simulink model "Simulation_Uncontrolled"  (R2020b)
settings: Solver=FixedStepAuto  StartTime=0.0  StopTime=8  FixedStep=0.01  RelTol=1e-3
undefined symbols (not defined in the file): sigbuilder_block
libraries: simulink x1
settings Model: Creator=Kacper  LastModifiedBy=Kacper

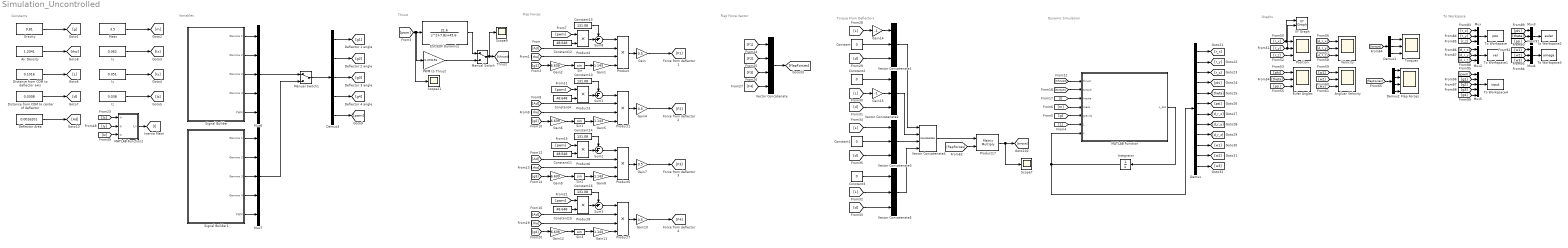
== system Simulation_Uncontrolled ==
  note: Graphs
  note: To Workspace
  note: Flap Force Vector
  note: Dynamic Simulation
  note: Torque From Deflectors
  note: Flap Forces
  note: Thrust
  note: Constants
  note: Variables
  Air Density : Constant  Value=1.2041
  Angluar Velocity : Scope  NumInputPorts=3
  Constant{,1..3} (4 alike) : Constant  Value=0
  Constant{10,13..14,16} (4 alike) : Constant  Value=131.08
  Constant{4,11..12,15} (4 alike) : Constant  Value=48.648
  Deflector Area : Constant  Value=0.0016201
  Demux : Demux  Outputs=12
  Demux1 : Demux  Outputs=3
  Demux2 : Demux
  Demux3 : Demux  Outputs=5
  Distance from COM to center of deflector : Constant  Value=0.0308
  Distance from COM to deflector axis : Constant  Value=0.1016
  ESC/EDF Dynamics : TransferFcn  Numerator=[21.6]  Denominator=[1 7.8 45.6]
  Euler Angles : Scope  NumInputPorts=3
  Flap Forces : Scope  NumInputPorts=4
  Gain{,4,7,10} (4 alike) : Gain  Gain=0.5
  Gain{1,5,8,11} (4 alike) : Gain  Gain=1.143
  Gain{2,6,9,12} (4 alike) : Gain  Gain=6.639
  Gain14 : Gain  Gain=-1
  Gain15 : Gain  Gain=-1
  Gravity : Constant  Value=9.81
  Integrator : Integrator  InitialCondition=[0;0;-0.6;deg2rad(0);deg2rad(0);deg2rad(0);0;0;0;0;0;0]
  Ix : Constant  Value=0.062
  Iy : Constant  Value=0.051
  Iz : Constant  Value=0.038
  MATLAB Function : MATLAB Function  TreatAsAtomicUnit=on
  MATLAB Function2 : MATLAB Function  TreatAsAtomicUnit=on
  Manual Switch : ManualSwitch
  Manual Switch1 : ManualSwitch
  Mass : Constant  Value=3.5
  Mux{,2..4} (4 alike) : Mux  Inputs=3
  Mux5 : Mux  Inputs=5
  Mux6 : Mux  Inputs=5
  Mux7 : Mux  Inputs=5
  PWM to Thrust : Gain  Gain=0.470193
  Position : Scope  NumInputPorts=3
  Product{,1,5,7} (4 alike) : Product  Inputs=4
  Product17 : Product  Multiplication=Matrix(*)
  Product{2..3,6,8} (4 alike) : Product
  Scope21 : Scope
  Scope7 : Scope
  Scope9 : Scope
  Signal Builder : Subsystem  Tag=STV Subsys  LoadFcn=sigbuilder_block('load');  StartFcn=sigbuilder_block('start');  StopFcn=sigbuilder_block('stop');  ClipboardFcn=sigbuilder_block('clipboard');  mask(Sigbuilder block){tuvar=[0:10]}
      mask help: Simulink:masks:SigbuilderBlock_MD
      mask init:
      | if ~strcmp(get_param(bdroot(gcbh),'SimulationStatus'),'stopped') tuvar = sigbuilder_block('maskInit'); end
      settings: CopyFcn=sigbuilder_block('copy');  DeleteFcn=sigbuilder_block('delete');  ModelCloseFcn=sigbuilder_block('modelClose');  PreSaveFcn=sigbuilder_block('preSave');  PauseFcn=sigbuilder_block('pause');  ContinueFcn=sigbuilder_block('continue');  NameChangeFcn=sigbuilder_block('namechange');  OpenFcn=sigbuilder_block('open',[6 22.5 1428 689.25 ]);  CloseFcn=sigbuilder_block('close');
      mask Display: plot(0, 0, 100, 100,[2, 2, 32, 32, 2], [68, 8, 8, 68, 68],[32, 2], [38, 38], [32, 19, 2],[53, 60, 44], [32, 17, 17, 2],[16, 16, 31, 31]);txt = getActiveGroup(gcbh);text(2, 100, txt,'verticalAlignment', 'top');
  Signal Builder1 : Subsystem  Tag=STV Subsys  LoadFcn=sigbuilder_block('load');  StartFcn=sigbuilder_block('start');  StopFcn=sigbuilder_block('stop');  ClipboardFcn=sigbuilder_block('clipboard');  mask(Sigbuilder block){tuvar=[0:10]}
      mask help: Simulink:masks:SigbuilderBlock_MD
      mask init:
      | if ~strcmp(get_param(bdroot(gcbh),'SimulationStatus'),'stopped') tuvar = sigbuilder_block('maskInit'); end
      settings: CopyFcn=sigbuilder_block('copy');  DeleteFcn=sigbuilder_block('delete');  ModelCloseFcn=sigbuilder_block('modelClose');  PreSaveFcn=sigbuilder_block('preSave');  PauseFcn=sigbuilder_block('pause');  ContinueFcn=sigbuilder_block('continue');  NameChangeFcn=sigbuilder_block('namechange');  OpenFcn=sigbuilder_block('open',[6 22.5 1428 689.25 ]);  CloseFcn=sigbuilder_block('close');
      mask Display: plot(0, 0, 100, 100,[2, 2, 32, 32, 2], [68, 8, 8, 68, 68],[32, 2], [38, 38], [32, 19, 2],[53, 60, 44], [32, 17, 17, 2],[16, 16, 31, 31]);txt = getActiveGroup(gcbh);text(2, 100, txt,'verticalAlignment', 'top');
  Sin{,1..3} (4 alike) : Trigonometry  ApproximationMethod=CORDIC
  Sum{1..3,8} (4 alike) : Sum  Inputs=-+|
  To Workspace : ToWorkspace  VariableName=pos  SaveFormat=Timeseries  SampleTime=-1
  To Workspace1 : ToWorkspace  VariableName=vel  SaveFormat=Timeseries  SampleTime=-1
  To Workspace2 : ToWorkspace  VariableName=euler  SaveFormat=Timeseries  SampleTime=-1
  To Workspace3 : ToWorkspace  VariableName=omega  SaveFormat=Timeseries  SampleTime=-1
  To Workspace4 : ToWorkspace  VariableName=input  SaveFormat=Timeseries  SampleTime=-1
  Torques : Scope  NumInputPorts=3
  Vector Concatenate : Concatenate  NumInputs=4
  Vector Concatenate{1..3,5} (4 alike) : Concatenate  NumInputs=3
  Vector Concatenate4 : Concatenate  NumInputs=4  Mode=Multidimensional array  ConcatenateDimension=2
  Velocity : Scope  NumInputPorts=3
  XY Graph : simulink/Sinks/XY Graph  xmin=-1  xmax=1  ymin=-1  ymax=1  st=-1
  wires:
  Gravity/1 -> [g]
  Mass/1 -> [m]
  Ix/1 -> [Ix]
  Iy/1 -> [Iy]
  Iz/1 -> [Iz]
  Distance from COM to deflector axis/1 -> [L]
  Distance from COM to center of deflector/1 -> [d]
  Air Density/1 -> [rho]
  Gain/1 -> [F1]
  Product/1 -> Gain/1
  [Ad] -> Product/2
  Product2/1 -> Sum8/2
  [rho] -> Product/3
  Gain2/1 -> Sin/1
  Sin/1 -> Gain1/1
  [pwm] -> Scope21/1, PWM to Thrust/1, ESC/EDF Dynamics/1
  ESC/EDF Dynamics/1 -> Manual Switch/1
  Constant12/1 -> Product2/2
  [pwm] -> Product2/1
  [F1] -> Vector Concatenate/1
  [F2] -> Vector Concatenate/2
  [F3] -> Vector Concatenate/3
  [F4] -> Vector Concatenate/4
  [L] -> Gain14/1
  [d] -> Vector Concatenate1/3
  Constant/1 -> Vector Concatenate1/2
  Gain14/1 -> Vector Concatenate1/1
  Gain15/1 -> Vector Concatenate2/2
  [L] -> Gain15/1
  Constant2/1 -> Vector Concatenate2/1
  Constant1/1 -> Vector Concatenate3/2
  [L] -> Vector Concatenate3/1
  [d] -> Vector Concatenate3/3
  Vector Concatenate1/1 -> Vector Concatenate4/1
  Vector Concatenate2/1 -> Vector Concatenate4/2
  Vector Concatenate3/1 -> Vector Concatenate4/3
  Vector Concatenate4/1 -> Product17/1
  Vector Concatenate/1 -> [flapForces]
  [d] -> Vector Concatenate2/3
  [d] -> Vector Concatenate5/3
  Constant3/1 -> Vector Concatenate5/1
  [L] -> Vector Concatenate5/2
  Vector Concatenate5/1 -> Vector Concatenate4/4
  Sum8/1 -> Product/1
  Constant13/1 -> Sum8/1
  MATLAB Function/1(x_dot) -> Integrator/1
  [L] -> MATLAB Function/6(L)
  [g] -> MATLAB Function/5(gravity)
  [m] -> MATLAB Function/4(mass)
  [I] -> MATLAB Function/3(Inertia)
  [torque] -> MATLAB Function/2(torque)
  [thrust] -> MATLAB Function/1(thrust)
  [Iy] -> MATLAB Function2/2(Iy)
  [Iz] -> MATLAB Function2/3(Iz)
  [Ix] -> MATLAB Function2/1(Ix)
  MATLAB Function2/1(I_v) -> [I]
  Demux/1 -> [r_x]
  Demux/2 -> [r_y]
  Demux/3 -> [r_z]
  Demux/4 -> [phi]
  Demux/5 -> [theta]
  Demux/6 -> [psi]
  Demux/7 -> [d_r_x]
  Demux/8 -> [d_r_y]
  Demux/9 -> [d_r_z]
  Demux/10 -> [w1]
  Demux/11 -> [w2]
  Demux/12 -> [w3]
  [r_y] -> XY Graph/2, Position/2
  [r_z] -> Position/3
  [phi] -> Euler Angles/1
  [theta] -> Euler Angles/2
  [psi] -> Euler Angles/3
  [d_r_x] -> Velocity/1
  [d_r_y] -> Velocity/2
  [d_r_z] -> Velocity/3
  [w1] -> Angluar Velocity/1
  [w2] -> Angluar Velocity/2
  [w3] -> Angluar Velocity/3
  [r_x] -> XY Graph/1, Position/1
  Demux1/1 -> Torques/1
  Demux1/2 -> Torques/2
  Demux1/3 -> Torques/3
  [torque] -> Demux1/1
  Demux2/1 -> Flap Forces/1
  Demux2/2 -> Flap Forces/2
  Demux2/3 -> Flap Forces/3
  Demux2/4 -> Flap Forces/4
  [flapForces] -> Demux2/1
  [flapForces] -> Product17/2
  Mux/1 -> To Workspace/1
  PWM to Thrust/1 -> Manual Switch/2
  Manual Switch/1 -> [thrust], Scope9/1
  [r_z] -> Mux/3
  [r_y] -> Mux/2
  [r_x] -> Mux/1
  [d_r_z] -> Mux2/3
  [d_r_x] -> Mux2/1
  Mux2/1 -> To Workspace1/1
  [d_r_y] -> Mux2/2
  [psi] -> Mux3/3
  [phi] -> Mux3/1
  Mux3/1 -> To Workspace2/1
  [theta] -> Mux3/2
  [w3] -> Mux4/3
  [w1] -> Mux4/1
  Mux4/1 -> To Workspace3/1
  [w2] -> Mux4/2
  [g2] -> Mux5/3
  [pwm] -> Mux5/1
  Mux5/1 -> To Workspace4/1
  [g1] -> Mux5/2
  [g3] -> Mux5/4
  [g4] -> Mux5/5
  Gain1/1 -> Product/4
  [g1] -> Gain2/1
  Deflector Area/1 -> [Ad]
  [Ad] -> Product1/2
  [rho] -> Product1/3
  Gain6/1 -> Sin1/1
  [g2] -> Gain6/1
  Constant10/1 -> Sum1/1
  [pwm] -> Product3/1
  Sum1/1 -> Product1/1
  Gain4/1 -> [F2]
  Gain5/1 -> Product1/4
  Product1/1 -> Gain4/1
  Product3/1 -> Sum1/2
  Sin1/1 -> Gain5/1
  Constant4/1 -> Product3/2
  [Ad] -> Product5/2
  [rho] -> Product5/3
  Gain9/1 -> Sin2/1
  [g3] -> Gain9/1
  Constant14/1 -> Sum2/1
  [pwm] -> Product6/1
  Sum2/1 -> Product5/1
  Gain7/1 -> [F3]
  Gain8/1 -> Product5/4
  Product5/1 -> Gain7/1
  Product6/1 -> Sum2/2
  Sin2/1 -> Gain8/1
  Constant11/1 -> Product6/2
  [Ad] -> Product7/2
  [rho] -> Product7/3
  Gain12/1 -> Sin3/1
  [g4] -> Gain12/1
  Constant16/1 -> Sum3/1
  [pwm] -> Product8/1
  Sum3/1 -> Product7/1
  Gain10/1 -> [F4]
  Gain11/1 -> Product7/4
  Product7/1 -> Gain10/1
  Product8/1 -> Sum3/2
  Sin3/1 -> Gain11/1
  Constant15/1 -> Product8/2
  Demux3/1 -> [g1]
  Integrator/1 -> Demux/1, MATLAB Function/7(x)
  Signal Builder/1(Gamma 1) -> Mux6/1
  Signal Builder/2(Gamma 2) -> Mux6/2
  Signal Builder/3(Gamma 3) -> Mux6/3
  Signal Builder/4(Gamma 4) -> Mux6/4
  Signal Builder/5(PWM) -> Mux6/5
  Signal Builder1/1(Gamma 1) -> Mux7/1
  Signal Builder1/2(Gamma 2) -> Mux7/2
  Signal Builder1/3(Gamma 3) -> Mux7/3
  Signal Builder1/4(Gamma 4) -> Mux7/4
  Signal Builder1/5(PWM) -> Mux7/5
  Demux3/2 -> [g2]
  Demux3/3 -> [g3]
  Demux3/4 -> [g4]
  Demux3/5 -> [pwm]
  Mux6/1 -> Manual Switch1/1
  Mux7/1 -> Manual Switch1/2
  Manual Switch1/1 -> Demux3/1
  Product17/1 -> Scope7/1, [torque]

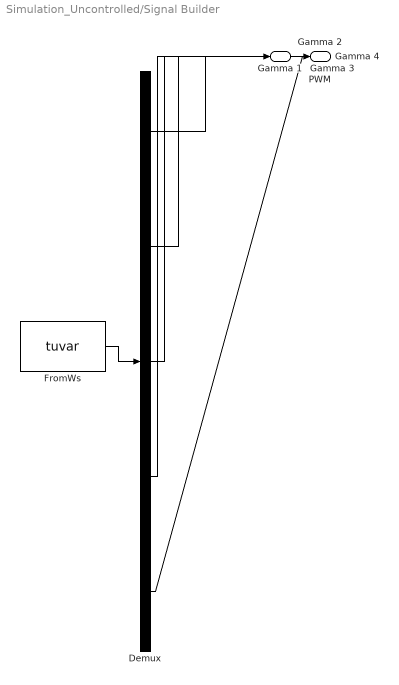
== system Simulation_Uncontrolled/Signal Builder ==
  Demux : Demux  Tag=STV Demux  Outputs=5
      settings: DisplayOption=none
  FromWs : FromWorkspace  Tag=STV FromWs  VariableName=tuvar
      SigBuilderData=|
      | common.afterFinalStr = 'Extrapolate'
      | common.sampleTime = 0
      | dataSet.timeRange = [0 20]
      | dataSet.name = 'First Simulation'
      | sbobj.Groups.Name = 'First Simulation'
      | sbobj.Groups.Signals(1).Name = 'Gamma 1'
      | sbobj.Groups.Signals(1).XData = [0 5 5 5.1 5.1 5.2 5.2 5.3 5.3 5.4 5.4 5.5 5.5 5.6 5.6 5.7 5.7 7 7 7.1 7.1 7.2 7.2 7.3 7.3 7.4 7.4 7.5 7.5 7.6 7.6 7.7 7.7 20]
      | sbobj.Groups.Signals(1).YData = [0 0 0.1745 0.1745 0 0 -0.1745 -0.1745 0 0 -0.1745 -0.1745 0 0 0.1745 0.1745 0 0 0.1745 0.1745 0 0 -0.1745 -0.1745 0 0 -0.1745 -0.1745 0 0 0.1745 0.1745 0 0]
      | sbobj.Groups.Signals(2).Name = 'Gamma 2'
      | sbobj.Groups.Signals(2).XData = [0 6 6 6.1 6.1 6.2 6.2 6.3 6.3 6.4 6.4 6.5 6.5 6.6 6.6 6.7 6.7 7 7 7.1 7.1 7.2 7.2 7.3 7.3 7.4 7.4 7.5 7.5 7.6 7.6 7.7 7.7 20]
      | sbobj.Groups.Signals(2).YData = [0 0 0.1745 0.1745 0 0 -0.1745 -0.1745 0 0 -0.1745 -0.1745 0 0 0.1745 0.1745 0 0 0.1745 0.1745 0 0 -0.1745 -0.1745 0 0 -0.1745 -0.1745 0 0 0.1745 0.1745 0 0]
      | sbobj.Groups.Signals(3).Name = 'Gamma 3'
      | sbobj.Groups.Signals(3).XData = [0 5 5 5.1 5.1 5.2 5.2 5.3 5.3 5.4 5.4 5.5 5.5 5.6 5.6 5.7 5.7 7 7 7.1 7.1 7.2 7.2 7.3 7.3 7.4 7.4 7.5 7.5 7.6 7.6 7.7 7.7 20]
      | sbobj.Groups.Signals(3).YData = [0 0 -0.1745 -0.1745 0 0 0.1745 0.1745 0 0 0.1745 0.1745 0 0 -0.1745 -0.1745 0 0 0.1745 0.1745 0 0 -0.1745 -0.1745 0 0 -0.1745 -0.1745 0 0 0.1745 0.1745 0 0]
      | sbobj.Groups.Signals(4).Name = 'Gamma 4'
      | sbobj.Groups.Signals(4).XData = [0 6 6 6.1 6.1 6.2 6.2 6.3 6.3 6.4 6.4 6.5 6.5 6.6 6.6 6.7 6.7 7 7 7.1 7.1 7.2 7.2 7.3 7.3 7.4 7.4 7.5 7.5 7.6 7.6 7.7 7.7 20]
      | sbobj.Groups.Signals(4).YData = [0 0 -0.1745 -0.1745 0 0 0.1745 0.1745 0 0 0.1745 0.1745 0 0 -0.1745 -0.1745 0 0 0.1745 0.1745 0 0 -0.1745 -0.1745 0 0 -0.1745 -0.1745 0 0 0.1745 0.1745 0 0]
      | sbobj.Groups.Signals(5).Name = 'PWM'
      | sbobj.Groups.Signals(5).XData = [0 1 2 2 3 3 4 4 20]
      | sbobj.Groups.Signals(5).YData = [90 75 75 90 90 60 60 71 71]
      | sbobj.Groups.TimeRange = [0 20]
  Gamma 1 : Outport  Tag=STV Outport
  Gamma 2 : Outport  Tag=STV Outport  Port=2
  Gamma 3 : Outport  Tag=STV Outport  Port=3
  Gamma 4 : Outport  Tag=STV Outport  Port=4
  PWM : Outport  Tag=STV Outport  Port=5
  wires:
  FromWs/1 -> Demux/1
  Demux/1 -> Gamma 1/1
  Demux/2 -> Gamma 2/1
  Demux/3 -> Gamma 3/1
  Demux/4 -> Gamma 4/1
  Demux/5 -> PWM/1

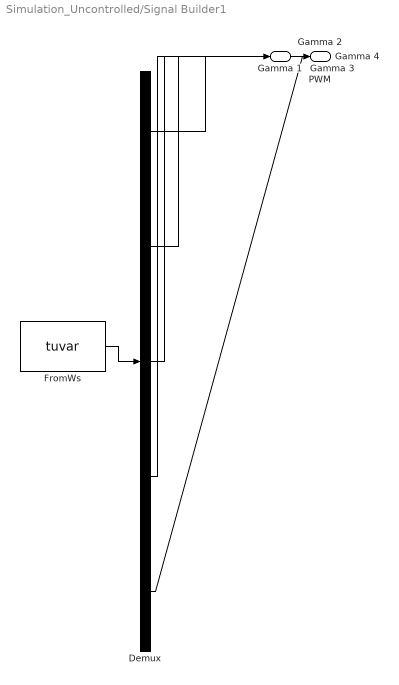
== system Simulation_Uncontrolled/Signal Builder1 ==
  Demux : Demux  Tag=STV Demux  Outputs=5
      settings: DisplayOption=none
  FromWs : FromWorkspace  Tag=STV FromWs  VariableName=tuvar
      SigBuilderData=|
      | common.afterFinalStr = 'Extrapolate'
      | common.sampleTime = 0
      | dataSet.timeRange = [0 8]
      | dataSet.name = 'Second Simulation'
      | sbobj.Groups.Name = 'Second Simulation'
      | sbobj.Groups.Signals(1).Name = 'Gamma 1'
      | sbobj.Groups.Signals(1).XData = [0 4.4 4.4 4.5 4.5 4.6 4.6 4.7 4.7 4.9 4.9 5 5 5.1 5.1 5.2 5.2 5.5 5.5 5.6 5.6 5.7 5.7 5.8 5.8 6 6 6.1 6.1 6.2 6.2 6.3 6.3 8]
      | sbobj.Groups.Signals(1).YData = [0 0 0.1745 0.1745 0 0 -0.1745 -0.1745 0 0 -0.1745 -0.1745 0 0 0.1745 0.1745 0 0 -0.1745 -0.1745 0 0 0.1745 0.1745 0 0 0.1745 0.1745 0 0 -0.1745 -0.1745 0 0]
      | sbobj.Groups.Signals(2).Name = 'Gamma 2'
      | sbobj.Groups.Signals(2).XData = [0 4.4 4.4 4.5 4.5 4.6 4.6 4.7 4.7 4.9 4.9 5 5 5.1 5.1 5.2 5.2 5.5 5.5 5.6 5.6 5.7 5.7 5.8 5.8 6 6 6.1 6.1 6.2 6.2 6.3 6.3 8]
      | sbobj.Groups.Signals(2).YData = [0 0 0.1745 0.1745 0 0 -0.1745 -0.1745 0 0 -0.1745 -0.1745 0 0 0.1745 0.1745 0 0 -0.1745 -0.1745 0 0 0.1745 0.1745 0 0 0.1745 0.1745 0 0 -0.1745 -0.1745 0 0]
      | sbobj.Groups.Signals(3).Name = 'Gamma 3'
      | sbobj.Groups.Signals(3).XData = [0 4.4 4.4 4.5 4.5 4.6 4.6 4.7 4.7 4.9 4.9 5 5 5.1 5.1 5.2 5.2 5.5 5.5 5.6 5.6 5.7 5.7 5.8 5.8 6 6 6.1 6.1 6.2 6.2 6.3 6.3 8]
      | sbobj.Groups.Signals(3).YData = [0 0 -0.1745 -0.1745 0 0 0.1745 0.1745 0 0 0.1745 0.1745 0 0 -0.1745 -0.1745 0 0 0.1745 0.1745 0 0 -0.1745 -0.1745 0 0 -0.1745 -0.1745 0 0 0.1745 0.1745 0 0]
      | sbobj.Groups.Signals(4).Name = 'Gamma 4'
      | sbobj.Groups.Signals(4).XData = [0 4.4 4.4 4.5 4.5 4.6 4.6 4.7 4.7 4.9 4.9 5 5 5.1 5.1 5.2 5.2 5.5 5.5 5.6 5.6 5.7 5.7 5.8 5.8 6 6 6.1 6.1 6.2 6.2 6.3 6.3 8]
      | sbobj.Groups.Signals(4).YData = [0 0 -0.1745 -0.1745 0 0 0.1745 0.1745 0 0 0.1745 0.1745 0 0 -0.1745 -0.1745 0 0 0.1745 0.1745 0 0 -0.1745 -0.1745 0 0 -0.1745 -0.1745 0 0 0.1745 0.1745 0 0]
      | sbobj.Groups.Signals(5).Name = 'PWM'
      | sbobj.Groups.Signals(5).XData = [0 1 2 3 4 8]
      | sbobj.Groups.Signals(5).YData = [90 75 75 75 75 75]
      | sbobj.Groups.TimeRange = [0 8]
  Gamma 1 : Outport  Tag=STV Outport
  Gamma 2 : Outport  Tag=STV Outport  Port=2
  Gamma 3 : Outport  Tag=STV Outport  Port=3
  Gamma 4 : Outport  Tag=STV Outport  Port=4
  PWM : Outport  Tag=STV Outport  Port=5
  wires:
  Demux/5 -> PWM/1
  Demux/4 -> Gamma 4/1
  Demux/3 -> Gamma 3/1
  Demux/2 -> Gamma 2/1
  Demux/1 -> Gamma 1/1
  FromWs/1 -> Demux/1

== matlab function Simulation_Uncontrolled/MATLAB Function ==
  data: thrust input; x_dot output; torque input; Inertia input; mass input; gravity input; L input; x input
function x_dot = dynamics(thrust,torque,Inertia,mass,gravity,L,x)
x_dot=zeros(12,1);
I = diag([Inertia(1,1),Inertia(2,2),Inertia(3,3)]);




phi = x(4);
theta = x(5);
psi = x(6);

omega = [x(10);x(11);x(12)]; 

omegaSkew = [0 -x(12) x(11);
             x(12) 0 x(10);
             -x(11) x(10) 0];

         
inv_H = [1 sin(phi)*tan(theta) cos(phi)*tan(theta);
         0 cos(phi) -sin(phi);
         0 sin(phi)/cos(theta) cos(phi)/cos(theta)];
     
R_b_to_e = [cos(theta)*cos(psi) cos(theta)*sin(psi) -sin(theta);
            sin(phi)*sin(theta)*cos(psi)-cos(phi)*sin(psi) sin(phi)*sin(theta)*sin(psi)+cos(phi)*cos(psi) sin(phi)*cos(theta)
            cos(phi)*sin(theta)*cos(psi)+sin(phi)*sin(psi) cos(phi)*sin(theta)*sin(psi)-sin(phi)*cos(psi) cos(phi)*cos(theta)];
        
thrustForce = [0;0;thrust];
gravityForce = [0;0;mass*gravity];
     
d_euler = inv_H * omega;

temp = (1/L)*R_b_to_e*torque;
dd_r = (1/mass)*(gravityForce - R_b_to_e * thrustForce + cross([0;0;1],temp));

d_omega = inv(I)*(-omegaSkew*I*omega + torque);

%[(cos(phi)*sin(psi)-cos(psi)*sin(phi)*sin(theta)), -(cos(phi)*cos(psi)+sin(phi)*sin(psi)*sin(theta)), -cos(theta)*sin(phi);
%cos(psi)*cos(theta), cos(theta)*sin(psi), -sin(theta);
%0, 0, 0]*torque;


x_dot(1) = x(7);
x_dot(2) = x(8);
x_dot(3) = x(9);

x_dot(4) = d_euler(1);
x_dot(5) = d_euler(2);
x_dot(6) = d_euler(3);

x_dot(7) = -dd_r(1);
x_dot(8) = -dd_r(2);
x_dot(9) = dd_r(3);

x_dot(10) = d_omega(1);
x_dot(11) = d_omega(2);
x_dot(12) = d_omega(3);

end

== matlab function Simulation_Uncontrolled/MATLAB Function2 ==
  data: Ix input; I_v output; Iy input; Iz input
function I_v = Inertia(Ix,Iy,Iz)
I_v = [Ix 0 0; 0 Iy 0; 0 0 Iz];
end
